simulink model "scheme2"  (R2024a)
settings: Solver=FixedStepDiscrete  StartTime=0.0  StopTime=10.0  FixedStep=10e-4  RelTol=1e-3
values from neighbouring files (symbols this model uses):
  a = 5    [main.m]
  b = 4    [main.m]
  c = 4    [main.m]
  k = par(1)    [main.m]
  T = par(2)    [main.m]
  w = logspace(-2, freq_domain_power, 1000)    [main.m]
undefined symbols (not defined in the file or in its folder): DiscIntNeverNeededParam
libraries: simulink x5
settings Model: Creator=alexivanov  LastModifiedBy=alexivanov

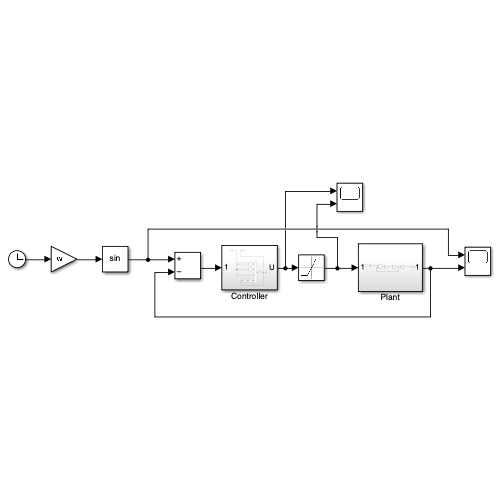
[thumbnail: Simulink's stored preview of the top-level diagram]
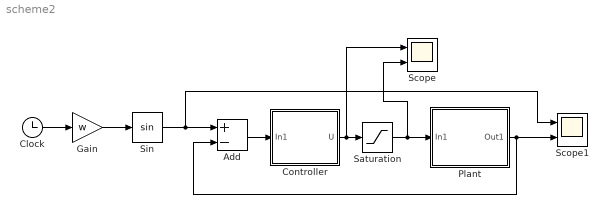
== system scheme2 ==
  Add : Sum  Inputs=+-
  Clock : Clock
      settings: Decimation=100
  Controller : Subsystem
  Gain : Gain  Gain=w
  Plant : Subsystem
  Saturation : Saturate
  Scope : Scope  NumInputPorts=2
  Scope1 : Scope  NumInputPorts=2
  Sin : Trigonometry
  wires:
  Gain/1 -> Sin/1
  Clock/1 -> Gain/1
  Sin/1 -> Scope1/1, Add/1
  Plant/1(Out1) -> Add/2, Scope1/2
  Add/1 -> Controller/1(In1)
  Controller/1(U) -> Saturation/1, Scope/1
  Saturation/1 -> Plant/1(In1), Scope/2

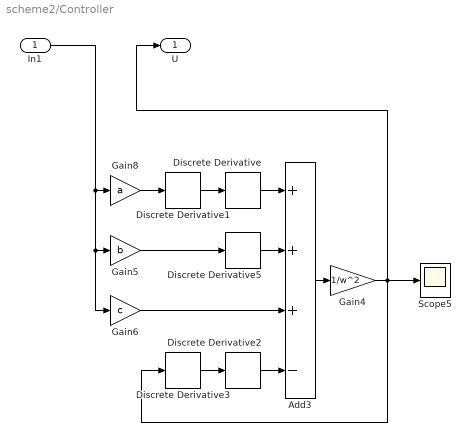
== system scheme2/Controller ==
  In1 : Inport
  Add3 : Sum  Inputs=+++-
  Discrete Derivative : simulink/Discrete/Discrete Derivative  gainval=1  ICPrevScaledInput=0.0  OutMin=[]  OutMax=[]  OutDataType=fixdt(1, 16)  OutScaling=2^-10  DoSatur=off
  Discrete Derivative{1..3,5} (4 alike) : simulink/Discrete/Discrete Derivative  gainval=1.0  ICPrevScaledInput=0.0  OutMin=[]  OutMax=[]  OutDataType=fixdt(1, 16)  OutScaling=2^-10  DoSatur=off
  Gain4 : Gain  Gain=1/w^2
  Gain5 : Gain  Gain=b
  Gain6 : Gain  Gain=c
  Gain8 : Gain  Gain=a
  Scope5 : Scope
  U : Outport
  wires:
  Gain6/1 -> Add3/3
  Gain5/1 -> Discrete Derivative5/1
  Discrete Derivative2/1 -> Add3/4
  Gain8/1 -> Discrete Derivative1/1
  Discrete Derivative3/1 -> Discrete Derivative2/1
  Add3/1 -> Gain4/1
  Gain4/1 -> U/1, Discrete Derivative3/1, Scope5/1
  In1/1 -> Gain6/1, Gain5/1, Gain8/1
  Discrete Derivative/1 -> Add3/1
  Discrete Derivative1/1 -> Discrete Derivative/1
  Discrete Derivative5/1 -> Add3/2

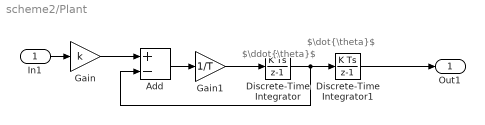
== system scheme2/Plant ==
  note: $\dot{\theta}$
  note: $\ddot{\theta}$
  In1 : Inport
  Add : Sum  Inputs=+-
  Discrete-Time Integrator : DiscreteIntegrator  SampleTime=-1  ICPrevOutput=DiscIntNeverNeededParam  ICPrevScaledInput=DiscIntNeverNeededParam
  Discrete-Time Integrator1 : DiscreteIntegrator  SampleTime=-1  ICPrevOutput=DiscIntNeverNeededParam  ICPrevScaledInput=DiscIntNeverNeededParam
  Gain : Gain  Gain=k
  Gain1 : Gain  Gain=1/T
  Out1 : Outport
  wires:
  In1/1 -> Gain/1
  Add/1 -> Gain1/1
  Discrete-Time Integrator1/1 -> Out1/1
  Gain/1 -> Add/1
  Discrete-Time Integrator/1 -> Add/2, Discrete-Time Integrator1/1
  Gain1/1 -> Discrete-Time Integrator/1
